simulink library "ilcDrag"  (R2022a)
settings: Solver=VariableStepAuto  StartTime=0.0  StopTime=10.0  RelTol=1e-3
undefined symbols (not defined in the file or in its folder): dragTurbine, env, hiLvlCtrl, thr, vhcl
libraries: calcFluidDynamicLoads x4, dspsigops x2, eulAng2RotMat_ul x1, linearLeastSqrs_ul x1, localApparentWind_ul x1, eeGeneralControl x1
settings Model: Creator=mcobb  LastModifiedBy=adabney
settings SolverCC: AlgebraicLoopSolver=TrustRegion
settings DebuggingCC: UnconnectedInputMsg=warning  UnconnectedOutputMsg=warning  UnconnectedLineMsg=warning  SFMachineParentedDataDiag=warning  ArithmeticOperatorsInVariantConditions=warning
settings SFSimCC: CustomCodeUndefinedFunction=UseInterfaceOnly

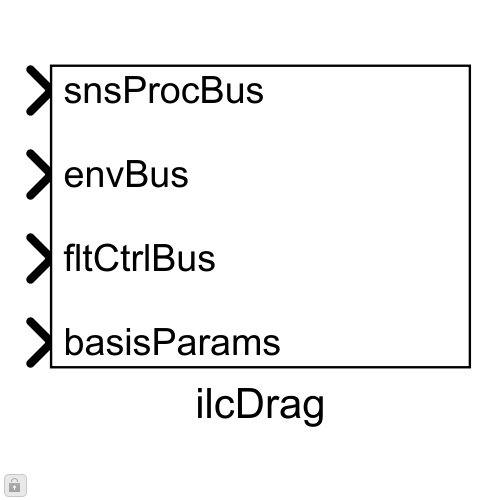
[thumbnail: Simulink's stored preview of the top-level diagram]
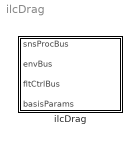
== system ilcDrag ==
  ilcDrag : Subsystem  mask{vhcl=vhcl, ctrl=hiLvlCtrl}
      mask prompts: vhcl "Vehicle Object"; ctrl "Controller Object"
      mask init:
      | S = vhcl.fluidRefArea.Value;
      | rho = 1000;
      settings: MinAlgLoopOccurrences=on
      mask DialogControl DescGroupVar Prompt: Iterative Learning Controller for Tether Drag
      mask DialogControl DescTextVar Prompt: Iterative learning controller which calculates a recursive least squares fit for the coefficient of tether drag. The parameterization is then used downstream to compute the desired AoA. Fit is also used to drive a physics based response surface.

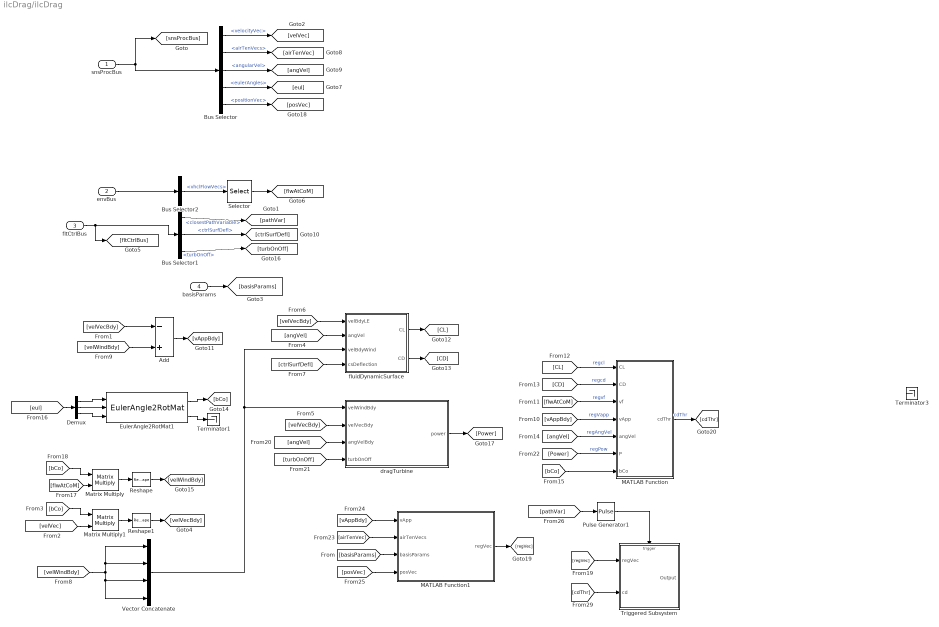
== system ilcDrag/ilcDrag ==
  snsProcBus : Inport  OutDataTypeStr=Bus: sensorsProcessingBus
  envBus : Inport  Port=2  OutDataTypeStr=Bus: envBus
  fltCtrlBus : Inport  Port=3  OutDataTypeStr=Bus: fltCtrlBus
  basisParams : Inport  Port=4
  Add : Sum  Inputs=-+
  Bus Selector : BusSelector  OutputSignals=velocityVec,airTenVecs,angularVel,eulerAngles,positionVec
  Bus Selector1 : BusSelector  OutputSignals=closestPathVariable,ctrlSurfDefl,turbOnOff
  Bus Selector2 : BusSelector  OutputSignals=vhclFlowVecs
  Demux : Demux  Outputs=3
  EulerAngle2RotMat1 : eulAng2RotMat_ul/EulerAngle2RotMat  SystemSampleTime=-1  VariantActivationTime=update diagram  Latency=0  AutoFrameSizeCalculation=off
  MATLAB Function : MATLAB Function  TreatAsAtomicUnit=on
  MATLAB Function1 : MATLAB Function  TreatAsAtomicUnit=on
  Matrix Multiply : Product  Multiplication=Matrix(*)
  Matrix Multiply1 : Product  Multiplication=Matrix(*)
  Pulse Generator1 : DiscretePulseGenerator  PulseType=Time based  TimeSource=Use external signal  Period=0.002  PulseWidth=50
  Reshape : Reshape  OutputDimensionality=Column vector (2-D)
  Reshape1 : Reshape  OutputDimensionality=Column vector (2-D)
  Selector : Selector  NumberOfDimensions=2  InputPortWidth=3  IndexOptions=Select all,Index vector (dialog)  Indices=[1 3],5  OutputSizes=1,1
  Terminator1 : Terminator
  Terminator3 : Terminator
  Triggered Subsystem : Subsystem  TreatAsAtomicUnit=on
  Vector Concatenate : Concatenate  NumInputs=4  Mode=Multidimensional array  ConcatenateDimension=2
  dragTurbine : Subsystem  AncestorBlock=dragTurbine/dragTurbine  TreatAsAtomicUnit=on  mask{vhcl=vhcl, thr=thr}
      mask prompts: vhcl "Vehicle Object"; thr "Tether Object"
  fluidDynamicSurface : Subsystem  mask{vcl=vhcl, fluidDensity=env.water.density.Value, fluidMomentArms=vhcl.fluidMomentArms.Value, fluidRefArea=vhcl.fluidRefArea.Value, wingTips=vhcl.wingTipPositions.Value}
      mask prompts: vcl "Vehicle object"; fluidDensity "Fluid density"; fluidMomentArms "Fluid Moment Arms"; fluidRefArea "Fluid Reference Area"; wingTips "Wing Tips"
      mask help:
      | Input must be an 1×N struct array with fields:
      |     refArea
      |     aeroCentPosVec
      |     spanUnitVec
      |     chordUnitVec
      |     CL
      |     CD
      |     alpha
      |     GainCL
      |     GainCD
      |
      | where N is the number of aerodynamic surfaces
      settings: MinAlgLoopOccurrences=on
  wires:
  snsProcBus/1 -> [snsProcBus], Bus Selector/1
  envBus/1 -> Bus Selector2/1
  fltCtrlBus/1 -> Bus Selector1/1, [fltCtrlBus]
  Bus Selector1/1 -> [pathVar]  "<closestPathVariable>"
  Bus Selector/1 -> [velVec]  "<velocityVec>"
  [velVecBdy] -> fluidDynamicSurface/1(velBdyLE)
  Bus Selector2/1 -> Selector/1  "<vhclFlowVecs>"
  Selector/1 -> [flwAtCoM]
  Bus Selector/3 -> [angVel]  "<angularVel>"
  Bus Selector/2 -> [airTenVec]  "<airTenVecs>"
  [angVel] -> fluidDynamicSurface/2(angVel)
  Bus Selector1/2 -> [ctrlSurfDefl]  "<ctrlSurfDefl>"
  [ctrlSurfDefl] -> fluidDynamicSurface/4(csDeflection)
  [velWindBdy] -> Add/2
  Add/1 -> [vAppBdy]
  [vAppBdy] -> MATLAB Function/4(vApp)  "regVapp"
  [flwAtCoM] -> MATLAB Function/3(vf)  "regvf"
  fluidDynamicSurface/1(CL) -> [CL]
  fluidDynamicSurface/2(CD) -> [CD]
  [CL] -> MATLAB Function/1(CL)  "regcl"
  [CD] -> MATLAB Function/2(CD)  "regcd"
  [angVel] -> MATLAB Function/5(angVel)  "regAngVel"
  Bus Selector/4 -> [eul]  "<eulerAngles>"
  [eul] -> Demux/1
  EulerAngle2RotMat1/2 -> Terminator1/1
  EulerAngle2RotMat1/1 -> [bCo]
  [flwAtCoM] -> Matrix Multiply/2
  [bCo] -> Matrix Multiply/1
  Matrix Multiply/1 -> Reshape/1
  [velVecBdy] -> dragTurbine/2(velVecBdy)
  [angVel] -> dragTurbine/3(angVelBdy)
  Bus Selector1/3 -> [turbOnOff]  "<turbOnOff>"
  [turbOnOff] -> dragTurbine/4(turbOnOff)
  dragTurbine/1(power) -> [Power]
  [Power] -> MATLAB Function/6(P)  "regPow"
  Bus Selector/5 -> [posVec]  "<positionVec>"
  [vAppBdy] -> MATLAB Function1/1(vApp)
  [posVec] -> MATLAB Function1/4(posVec)
  [airTenVec] -> MATLAB Function1/2(airTenVecs)
  [basisParams] -> MATLAB Function1/3(basisParams)
  MATLAB Function1/1(regVec) -> [regVec]
  basisParams/1 -> [basisParams]
  Demux/2 -> EulerAngle2RotMat1/2
  Demux/1 -> EulerAngle2RotMat1/1
  Demux/3 -> EulerAngle2RotMat1/3
  Vector Concatenate/1 -> fluidDynamicSurface/3(velBdyWind), dragTurbine/1(velWindBdy)
  [velWindBdy] -> Vector Concatenate/2, Vector Concatenate/1, Vector Concatenate/3, Vector Concatenate/4
  Reshape/1 -> [velWindBdy]
  Matrix Multiply1/1 -> Reshape1/1
  [velVec] -> Matrix Multiply1/2
  [bCo] -> Matrix Multiply1/1
  Reshape1/1 -> [velVecBdy]
  [velVecBdy] -> Add/1
  [bCo] -> MATLAB Function/7(bCo)
  [regVec] -> Triggered Subsystem/1(regVec)
  Pulse Generator1/1 -> Triggered Subsystem/Trigger
  [pathVar] -> Pulse Generator1/1
  [cdThr] -> Triggered Subsystem/2(cd)
  MATLAB Function/1(cdThr) -> [cdThr]  "cdThr"

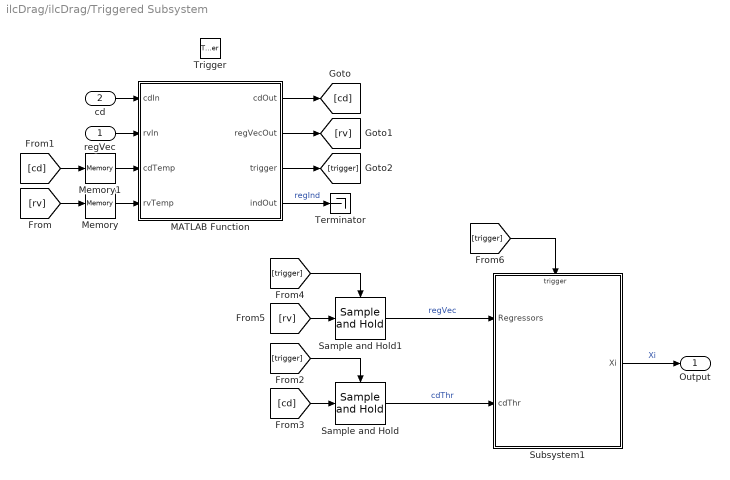
== system ilcDrag/ilcDrag/Triggered Subsystem ==
  regVec : Inport
  cd : Inport  Port=2
  Trigger : TriggerPort  VariantControl=(inherit)
  MATLAB Function : MATLAB Function  TreatAsAtomicUnit=on
  Memory : Memory  InitialCondition=zeros(500,10)  InheritSampleTime=on
  Memory1 : Memory  InitialCondition=zeros(500,1)  InheritSampleTime=on
  Sample and Hold : dspsigops/Sample and Hold  trig=Rising edge  initCond=zeros(500,1)  latchinput=off
  Sample and Hold1 : dspsigops/Sample and Hold  trig=Rising edge  initCond=zeros(500,10)  latchinput=off
  Subsystem1 : Subsystem
  Terminator : Terminator
  Output : Outport
  wires:
  regVec/1 -> MATLAB Function/2(rvIn)
  cd/1 -> MATLAB Function/1(cdIn)
  MATLAB Function/1(cdOut) -> [cd]
  Memory/1 -> MATLAB Function/4(rvTemp)
  Memory1/1 -> MATLAB Function/3(cdTemp)
  MATLAB Function/2(regVecOut) -> [rv]
  MATLAB Function/3(trigger) -> [trigger]
  [rv] -> Memory/1
  [cd] -> Memory1/1
  [trigger] -> Sample and Hold/Trigger
  [cd] -> Sample and Hold/1
  [trigger] -> Sample and Hold1/Trigger
  [rv] -> Sample and Hold1/1
  Subsystem1/1(Xi) -> Output/1  "Xi"
  [trigger] -> Subsystem1/Trigger
  Sample and Hold1/1 -> Subsystem1/1(Regressors)  "regVec"
  Sample and Hold/1 -> Subsystem1/2(cdThr)  "cdThr"
  MATLAB Function/4(indOut) -> Terminator/1  "regInd"

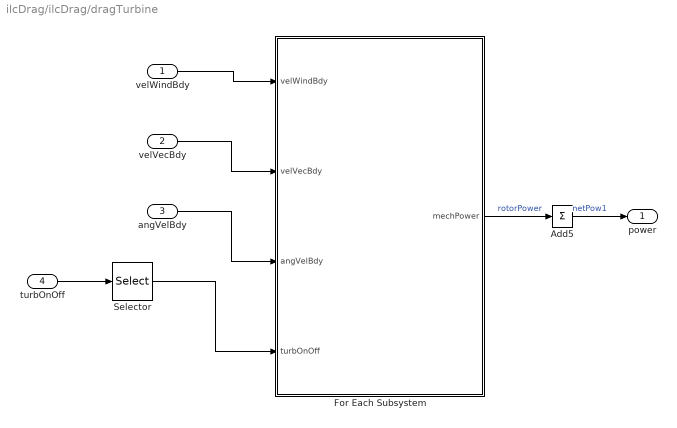
== system ilcDrag/ilcDrag/dragTurbine ==
  velWindBdy : Inport
  velVecBdy : Inport  Port=2
  angVelBdy : Inport  Port=3
  turbOnOff : Inport  Port=4
  Add5 : Sum  Inputs=1  CollapseDim=2
  For Each Subsystem : Subsystem  TreatAsAtomicUnit=on  mask{rho=rho, turb_struct=vhcl.struct('OCT.turb'), vhcl=vhcl}
      mask prompts: rho "Fluid Density"; turb_struct "Turbine Structure"; vhcl "Vehicle"
  Selector : Selector  InputPortWidth=1+vhcl.numTurbines.Value  IndexOptions=Index vector (dialog)  Indices=1  OutputSizes=1
  power : Outport  PortDimensions=[1,1]  VectorParamsAs1DForOutWhenUnconnected=off
  wires:
  Selector/1 -> For Each Subsystem/4(turbOnOff)
  Add5/1 -> power/1  "netPow1"
  velWindBdy/1 -> For Each Subsystem/1(velWindBdy)
  turbOnOff/1 -> Selector/1
  angVelBdy/1 -> For Each Subsystem/3(angVelBdy)
  velVecBdy/1 -> For Each Subsystem/2(velVecBdy)
  For Each Subsystem/1(mechPower) -> Add5/1  "rotorPower"

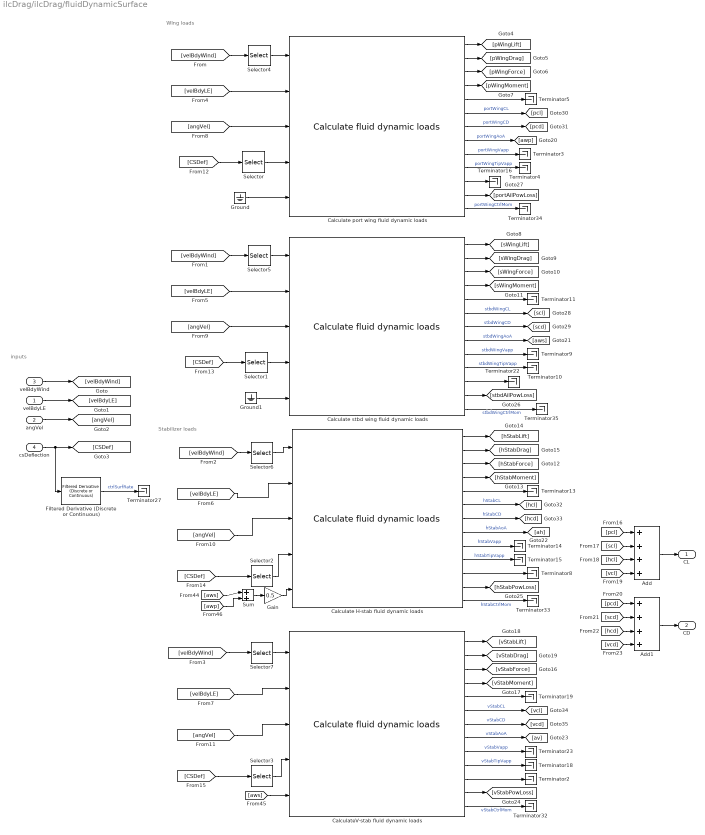
== system ilcDrag/ilcDrag/fluidDynamicSurface ==
  note: inputs
  note: Stabilizer loads
  note: WIng loads
  velBdyLE : Inport
  angVel : Inport  Port=2
  velBdyWind : Inport  Port=3
  csDeflection : Inport  Port=4
  Add : Sum  Inputs=++++
  Add1 : Sum  Inputs=++++
  Calculate H-stab fluid dynamic loads : calcFluidDynamicLoads/Calculate fluid dynamic loads  aSurf=vcl.hStab  sRef=fluidRefArea  rArm_LE=fluidMomentArms(:,3)  rTip_LE=wingTips(:,3)  fluidDensity=fluidDensity
  Calculate port wing fluid dynamic loads : calcFluidDynamicLoads/Calculate fluid dynamic loads  aSurf=vcl.portWing  sRef=fluidRefArea  rArm_LE=fluidMomentArms(:,1)  rTip_LE=wingTips(:,1)  fluidDensity=fluidDensity
  Calculate stbd wing fluid dynamic loads : calcFluidDynamicLoads/Calculate fluid dynamic loads  aSurf=vcl.stbdWing  sRef=fluidRefArea  rArm_LE=fluidMomentArms(:,2)  rTip_LE=wingTips(:,2)  fluidDensity=fluidDensity
  CalculateV-stab fluid dynamic loads : calcFluidDynamicLoads/Calculate fluid dynamic loads  aSurf=vcl.vStab  sRef=fluidRefArea  rArm_LE=fluidMomentArms(:,4)  rTip_LE=wingTips(:,4)  fluidDensity=fluidDensity
  Filtered Derivative (Discrete or Continuous) : eeGeneralControl/Filtered Derivative (Discrete or Continuous)  K=1  T=.001  B=inf  A=-inf  minRatio=10  init_option=Inherited from block input  x0=0  Ts=-1
      settings: SourceProductBaseCode=PS
  Gain : Gain  Gain=0.5
  Ground : Ground
  Ground1 : Ground
  Selector : Selector  InputPortWidth=4  IndexOptions=Index vector (dialog)  Indices=1  OutputSizes=1
  Selector1 : Selector  InputPortWidth=4  IndexOptions=Index vector (dialog)  Indices=2  OutputSizes=1
  Selector2 : Selector  InputPortWidth=4  IndexOptions=Index vector (dialog)  Indices=3  OutputSizes=1
  Selector3 : Selector  InputPortWidth=4  IndexOptions=Index vector (dialog)  Indices=4  OutputSizes=1
  Selector4 : Selector  NumberOfDimensions=2  InputPortWidth=4  IndexOptions=Select all,Index vector (dialog)  Indices=1,1  OutputSizes=1,1
  Selector5 : Selector  NumberOfDimensions=2  InputPortWidth=4  IndexOptions=Select all,Index vector (dialog)  Indices=1,2  OutputSizes=1,1
  Selector6 : Selector  NumberOfDimensions=2  InputPortWidth=4  IndexOptions=Select all,Index vector (dialog)  Indices=1,3  OutputSizes=1,1
  Selector7 : Selector  NumberOfDimensions=2  InputPortWidth=4  IndexOptions=Select all,Index vector (dialog)  Indices=1,4  OutputSizes=1,1
  Sum : Sum  Inputs=|++
  Terminator{2..5,8..11,13..16,18..19,22..23,27,32..35} (21 alike) : Terminator
  CL : Outport
  CD : Outport  Port=2
  wires:
  Ground1/1 -> Calculate stbd wing fluid dynamic loads/5
  Ground/1 -> Calculate port wing fluid dynamic loads/5
  Sum/1 -> Gain/1
  Gain/1 -> Calculate H-stab fluid dynamic loads/5
  [awp] -> Sum/2
  [aws] -> Sum/1
  [aws] -> CalculateV-stab fluid dynamic loads/5
  Calculate stbd wing fluid dynamic loads/13 -> Terminator35/1  "stbdWingCtrlMom"
  Calculate port wing fluid dynamic loads/13 -> Terminator34/1  "portWingCtrlMom"
  Calculate H-stab fluid dynamic loads/13 -> Terminator33/1  "hStabCtrlMom"
  CalculateV-stab fluid dynamic loads/13 -> Terminator32/1  "vStabCtrlMom"
  Filtered Derivative (Discrete or Continuous)/1 -> Terminator27/1  "ctrlSurfRate"
  Calculate port wing fluid dynamic loads/12 -> [portAilPowLoss]
  Calculate stbd wing fluid dynamic loads/12 -> [stbdAilPowLoss]
  Calculate H-stab fluid dynamic loads/12 -> [hStabPowLoss]
  CalculateV-stab fluid dynamic loads/12 -> [vStabPowLoss]
  CalculateV-stab fluid dynamic loads/11 -> Terminator2/1
  Calculate H-stab fluid dynamic loads/11 -> Terminator8/1
  Calculate stbd wing fluid dynamic loads/11 -> Terminator22/1
  Calculate port wing fluid dynamic loads/11 -> Terminator16/1
  Selector7/1 -> CalculateV-stab fluid dynamic loads/1
  Selector6/1 -> Calculate H-stab fluid dynamic loads/1
  Selector5/1 -> Calculate stbd wing fluid dynamic loads/1
  Selector4/1 -> Calculate port wing fluid dynamic loads/1
  CalculateV-stab fluid dynamic loads/7 -> [vcd]  "vStabCD"
  CalculateV-stab fluid dynamic loads/10 -> Terminator18/1  "vStabTipVapp"
  CalculateV-stab fluid dynamic loads/2 -> [vStabDrag]
  CalculateV-stab fluid dynamic loads/5 -> Terminator19/1
  CalculateV-stab fluid dynamic loads/8 -> [av]  "vStabAoA"
  CalculateV-stab fluid dynamic loads/4 -> [vStabMoment]
  CalculateV-stab fluid dynamic loads/9 -> Terminator23/1  "vStabVapp"
  CalculateV-stab fluid dynamic loads/6 -> [vcl]  "vStabCL"
  CalculateV-stab fluid dynamic loads/1 -> [vStabLift]
  CalculateV-stab fluid dynamic loads/3 -> [vStabForce]
  Calculate H-stab fluid dynamic loads/9 -> Terminator14/1  "hStabVapp"
  Calculate H-stab fluid dynamic loads/10 -> Terminator15/1  "hStabTipVapp"
  Calculate H-stab fluid dynamic loads/8 -> [ah]  "hStabAoA"
  Calculate H-stab fluid dynamic loads/3 -> [hStabForce]
  Calculate H-stab fluid dynamic loads/6 -> [hcl]  "hStabCL"
  Calculate H-stab fluid dynamic loads/1 -> [hStabLift]
  Calculate H-stab fluid dynamic loads/7 -> [hcd]  "hStabCD"
  Calculate H-stab fluid dynamic loads/5 -> Terminator13/1
  Calculate H-stab fluid dynamic loads/4 -> [hStabMoment]
  Calculate H-stab fluid dynamic loads/2 -> [hStabDrag]
  Calculate stbd wing fluid dynamic loads/4 -> [sWingMoment]
  Calculate stbd wing fluid dynamic loads/3 -> [sWingForce]
  Calculate stbd wing fluid dynamic loads/2 -> [sWingDrag]
  Calculate stbd wing fluid dynamic loads/1 -> [sWingLift]
  Calculate stbd wing fluid dynamic loads/10 -> Terminator10/1  "stbdWingTipVapp"
  Calculate stbd wing fluid dynamic loads/7 -> [scd]  "stbdWingCD"
  Calculate stbd wing fluid dynamic loads/8 -> [aws]  "stbdWingAoA"
  Calculate stbd wing fluid dynamic loads/6 -> [scl]  "stbdWingCL"
  Calculate stbd wing fluid dynamic loads/9 -> Terminator9/1  "stbdWingVapp"
  Calculate stbd wing fluid dynamic loads/5 -> Terminator11/1
  Calculate port wing fluid dynamic loads/5 -> Terminator5/1
  Calculate port wing fluid dynamic loads/10 -> Terminator4/1  "portWingTipVapp"
  Calculate port wing fluid dynamic loads/9 -> Terminator3/1  "portWingVapp"
  Calculate port wing fluid dynamic loads/8 -> [awp]  "portWingAoA"
  Calculate port wing fluid dynamic loads/7 -> [pcd]  "portWingCD"
  Calculate port wing fluid dynamic loads/6 -> [pcl]  "portWingCL"
  Calculate port wing fluid dynamic loads/4 -> [pWingMoment]
  Calculate port wing fluid dynamic loads/3 -> [pWingForce]
  Calculate port wing fluid dynamic loads/2 -> [pWingDrag]
  Calculate port wing fluid dynamic loads/1 -> [pWingLift]
  Selector3/1 -> CalculateV-stab fluid dynamic loads/4
  Selector2/1 -> Calculate H-stab fluid dynamic loads/4
  [CSDef] -> Selector3/1
  [CSDef] -> Selector2/1
  [CSDef] -> Selector1/1
  Selector1/1 -> Calculate stbd wing fluid dynamic loads/4
  Selector/1 -> Calculate port wing fluid dynamic loads/4
  [CSDef] -> Selector/1
  [angVel] -> CalculateV-stab fluid dynamic loads/3
  [angVel] -> Calculate H-stab fluid dynamic loads/3
  [angVel] -> Calculate stbd wing fluid dynamic loads/3
  [angVel] -> Calculate port wing fluid dynamic loads/3
  [velBdyLE] -> CalculateV-stab fluid dynamic loads/2
  [velBdyLE] -> Calculate H-stab fluid dynamic loads/2
  [velBdyLE] -> Calculate stbd wing fluid dynamic loads/2
  [velBdyLE] -> Calculate port wing fluid dynamic loads/2
  [velBdyWind] -> Selector7/1
  [velBdyWind] -> Selector6/1
  [velBdyWind] -> Selector5/1
  [velBdyWind] -> Selector4/1
  csDeflection/1 -> [CSDef], Filtered Derivative (Discrete or Continuous)/1
  velBdyWind/1 -> [velBdyWind]
  velBdyLE/1 -> [velBdyLE]
  angVel/1 -> [angVel]
  [pcl] -> Add/1
  [vcl] -> Add/4
  [hcl] -> Add/3
  [scl] -> Add/2
  Add/1 -> CL/1
  [pcd] -> Add1/1
  [vcd] -> Add1/4
  Add1/1 -> CD/1
  [hcd] -> Add1/3
  [scd] -> Add1/2

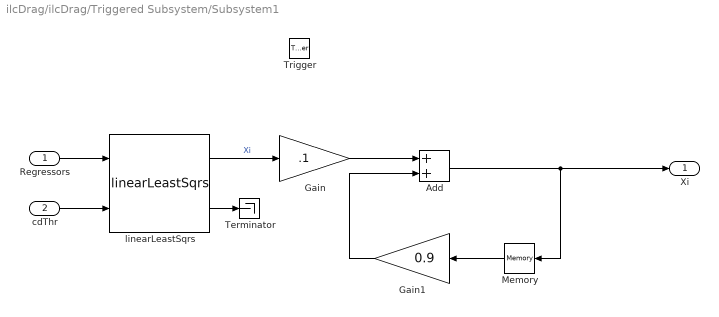
== system ilcDrag/ilcDrag/Triggered Subsystem/Subsystem1 ==
  Regressors : Inport
  cdThr : Inport  Port=2
  Trigger : TriggerPort  VariantControl=(inherit)  PortDimensions=1
  Add : Sum
  Gain : Gain  Gain=.1
  Gain1 : Gain  Gain=0.9
  Memory : Memory  InitialCondition=zeros(10,1)  InheritSampleTime=on
  Terminator : Terminator
  linearLeastSqrs : linearLeastSqrs_ul/linearLeastSqrs  SystemSampleTime=-1  VariantActivationTime=update diagram  Latency=0  AutoFrameSizeCalculation=off
  Xi : Outport
  wires:
  Regressors/1 -> linearLeastSqrs/1
  cdThr/1 -> linearLeastSqrs/2
  linearLeastSqrs/1 -> Gain/1  "Xi"
  Gain/1 -> Add/1
  Add/1 -> Xi/1, Memory/1
  Gain1/1 -> Add/2
  Memory/1 -> Gain1/1
  linearLeastSqrs/2 -> Terminator/1

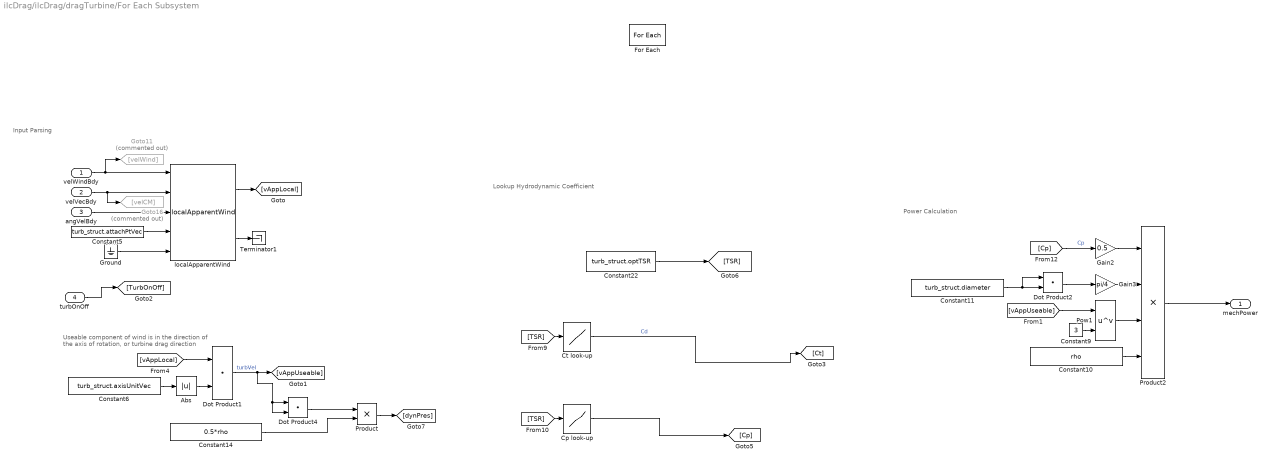
== system ilcDrag/ilcDrag/dragTurbine/For Each Subsystem ==
  note: Useable component of wind is in the direction of
      | the axis of rotation, or turbine drag direction
  note: Power Calculation
  note: Input Parsing
  note: Lookup Hydrodynamic Coefficient
  velWindBdy : Inport  Partition=on  PartitionDimension=2  PartitionWidth=1  PartitionOffset=0
  velVecBdy : Inport  Port=2
  angVelBdy : Inport  Port=3
  turbOnOff : Inport  Port=4
  Abs : Abs  SaturateOnIntegerOverflow=off
  Constant10 : Constant  Value=rho
  Constant11 : Constant  Value=turb_struct.diameter  VectorParams1D=off
  Constant14 : Constant  Value=0.5*rho
  Constant22 : Constant  Value=turb_struct.optTSR
  Constant5 : Constant  Value=turb_struct.attachPtVec
  Constant6 : Constant  Value=turb_struct.axisUnitVec
  Constant9 : Constant  Value=3
  Cp look-up : Lookup_n-D  NumberOfTableDimensions=1  BreakpointsForDimension1=turb_struct.RPMref  Table=turb_struct.CpLookup  InternalRulePriority=Speed  RndMeth=Simplest
  Ct look-up : Lookup_n-D  NumberOfTableDimensions=1  BreakpointsForDimension1=turb_struct.RPMref  Table=turb_struct.CtLookup  InternalRulePriority=Speed  RndMeth=Simplest
  Dot Product1 : DotProduct  OutDataTypeStr=Inherit: Inherit via internal rule
  Dot Product2 : DotProduct  OutDataTypeStr=Inherit: Inherit via internal rule
  Dot Product4 : DotProduct  OutDataTypeStr=Inherit: Inherit via internal rule
  For Each : ForEach  DisableCoverage=on  IterateSubsysMaskParameter=off,on,off  SubsysMaskParameterIterationDimension=1,2,1  SubsysMaskParameterIterationStepSize=1,1,1
  Gain2 : Gain  Gain=0.5
  Gain3 : Gain  Gain=pi/4
  Goto11 : Goto  Commented=on  GotoTag=velWind
  Goto16 : Goto  Commented=on  GotoTag=velCM
  Ground : Ground
  Pow1 : Math  Operator=pow  SignedPower=on  RndMeth=Zero
  Product : Product
  Product2 : Product  Inputs=4
  Terminator1 : Terminator
  localApparentWind : localApparentWind_ul/localApparentWind  SystemSampleTime=-1  VariantActivationTime=update diagram  Latency=0  AutoFrameSizeCalculation=off
  mechPower : Outport  PortDimensions=[1,1]  ConcatenationDimension=2  VectorParamsAs1DForOutWhenUnconnected=off
  wires:
  Constant22/1 -> [TSR]
  velWindBdy/1 -> Goto11/1, localApparentWind/1
  Dot Product1/1 -> [vAppUseable], Dot Product4/2, Dot Product4/1  "turbVel"
  Ground/1 -> localApparentWind/5
  Product/1 -> [dynPres]
  Constant14/1 -> Product/2
  velVecBdy/1 -> Goto16/1, localApparentWind/2
  [TSR] -> Cp look-up/1
  Abs/1 -> Dot Product1/2
  [Cp] -> Gain2/1  "Cp"
  localApparentWind/2 -> Terminator1/1
  Constant5/1 -> localApparentWind/4
  localApparentWind/1 -> [vAppLocal]
  Constant6/1 -> Abs/1
  Constant9/1 -> Pow1/2
  Pow1/1 -> Product2/3
  Dot Product4/1 -> Product/1
  Product2/1 -> mechPower/1
  turbOnOff/1 -> [TurbOnOff]
  Gain3/1 -> Product2/2
  Cp look-up/1 -> [Cp]
  [vAppLocal] -> Dot Product1/1
  Dot Product2/1 -> Gain3/1
  [vAppUseable] -> Pow1/1
  Constant10/1 -> Product2/4
  [TSR] -> Ct look-up/1
  Constant11/1 -> Dot Product2/1, Dot Product2/2
  angVelBdy/1 -> localApparentWind/3
  Gain2/1 -> Product2/1
  Ct look-up/1 -> [Ct]  "Cd"

== matlab function ilcDrag/MATLAB Function1 ==
  data: vApp input; regVec output; airTenVecs input; basisParams input; posVec input
function regVec = formRegVec(vApp,airTenVecs,basisParams, posVec)
regVec = zeros(1,10);
vAppMag = sqrt(sum(vApp.^2));
tenMag = sqrt(sum(airTenVecs.^2));
tanTheta = airTenVecs(3)/airTenVecs(1);

vApp = reshape(vApp,[1,3]);

el = basisParams(3);
cEl = cos(el);
sEl = sin(el);
thr = basisParams(5);

rotMat = [cEl 0 -sEl;0 1 0;sEl 0 cEl];
pos1 = rotMat'*posVec;


regVec(1) = pos1(2);
regVec(2) = pos1(3);
regVec(3) = posVec(3); 
regVec(4) = thr(1);
regVec(5) = vApp(1);
regVec(6) = vApp(2);
regVec(7) = vApp(3);
regVec(8) = vAppMag(1);
regVec(9) = tenMag(1);
regVec(10) = tanTheta(1);

== matlab function ilcDrag/MATLAB Function ==
  data: CL input; cdThr output; CD input; vf input; vApp input; angVel input; P input; bCo input
function cdThr = fcn(CL,CD,vf,vApp,angVel,P,bCo)

CD = sqrt(sum(CD.^2));
CL = sqrt(sum(CL.^2));

rho = 1000; %[kg/m^3]
% vFlowMag = sqrt(sum(vf.^2));
vAppMag = sqrt(sum(vApp.^2));

portR = -1.6667; %[m]
eta = angVel(3)*portR/vAppMag;

d = 1;
S = 9;
cp = 0.317*pi*(d/2)^2/S;
ct = 0.470*pi*(d/2)^2/S;

k = bCo(3,:);
vFlowMag = abs(dot(k,vf));

cpEff = 2*cp*((1+eta).^3+(1-eta).^3);
ctEff = 2*ct*((1+eta).^2+(1-eta).^2);

cdThr = zeros(1,1);
cdThr = (1/2*rho*vFlowMag^3*S*CL^3*cpEff/P)^(1/3)-CD-ctEff;

== matlab function ilcDrag/Triggered Subsystem/MATLAB Function ==
  data: cdIn input; cdOut output; rvIn input; cdTemp input; rvTemp input; regVecOut output; trigger output; indOut output
function [cdOut,regVecOut,trigger,indOut] = fcn(cdIn,rvIn,cdTemp,rvTemp)

ind = find(cdTemp == 0,1,'first');

cdOut = cdTemp;
regVecOut = rvTemp;

if ~isempty(ind)
    cdOut(ind) = cdIn;
    regVecOut(ind,:) = rvIn;
else
    cdOut(~ind) = 0;
    cdOut(1) = cdIn;
    regVecOut(~ind,:) = 0;
    regVecOut(1,:) = rvIn;
    ind = 1;
end
indOut = ind(1);
trigger = (ind(1)==500);
